simulink model "interrupt_gen"  (R2020a)
settings: Solver=FixedStepDiscrete  StartTime=0.0  StopTime=10.0  FixedStep=0.5  RelTol=1e-3
settings Model: Creator=sunip  LastModifiedBy=sunip
settings OptimizationCC: BlockReduction=off  ConditionallyExecuteInputs=off  DefaultParameterBehavior=Inlined
settings DebuggingCC: AlgebraicLoopMsg=error
settings HardwareCC: ProdBitPerPointer=32  ProdBitPerSizeT=32  ProdBitPerPtrDiffT=32  ProdLargestAtomicFloat=None  ProdIntDivRoundTo=Undefined  ProdEndianess=Unspecified  ProdWordSize=32  ProdHWDeviceType=ASIC/FPGA->ASIC/FPGA  TargetBitPerLong=64  TargetBitPerPointer=64  TargetBitPerSizeT=64  TargetBitPerPtrDiffT=64  TargetLongLongMode=on  TargetIntDivRoundTo=Zero  TargetEndianess=LittleEndian  TargetWordSize=64  TargetHWDeviceType=Custom Processor->MATLAB Host Computer  ProdEqTarget=off

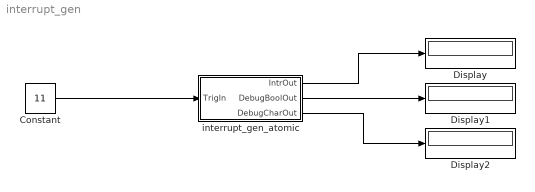
== system interrupt_gen ==
  Constant : Constant  Value=11  OutDataTypeStr=uint8  SampleTime=-1
  Display : Display
  Display1 : Display
  Display2 : Display
  interrupt_gen_atomic : Subsystem  TreatAsAtomicUnit=on
  wires:
  interrupt_gen_atomic/1(IntrOut) -> Display/1
  Constant/1 -> interrupt_gen_atomic/1(TrigIn)
  interrupt_gen_atomic/2(DebugBoolOut) -> Display1/1
  interrupt_gen_atomic/3(DebugCharOut) -> Display2/1

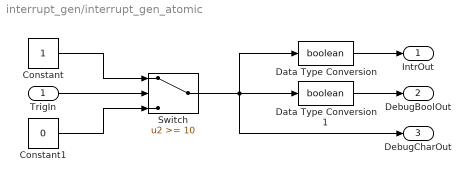
== system interrupt_gen/interrupt_gen_atomic ==
  TrigIn : Inport  OutDataTypeStr=uint8
  Constant : Constant  OutDataTypeStr=uint8  SampleTime=-1
  Constant1 : Constant  Value=0  OutDataTypeStr=uint8  SampleTime=-1
  Data Type Conversion : DataTypeConversion  OutDataTypeStr=boolean
  Data Type Conversion1 : DataTypeConversion  OutDataTypeStr=boolean
  Switch : Switch  Threshold=10  OutDataTypeStr=uint8
  IntrOut : Outport  OutDataTypeStr=boolean
  DebugBoolOut : Outport  Port=2  OutDataTypeStr=boolean
  DebugCharOut : Outport  Port=3
  wires:
  TrigIn/1 -> Switch/2
  Switch/1 -> DebugCharOut/1, Data Type Conversion1/1, Data Type Conversion/1
  Constant/1 -> Switch/1
  Constant1/1 -> Switch/3
  Data Type Conversion/1 -> IntrOut/1
  Data Type Conversion1/1 -> DebugBoolOut/1
